simulink model "lab6_splp"  (R2023b)
settings: Solver=ode23t  StartTime=0.0  StopTime=Tmdl  MaxStep=1e-4  RelTol=1e-3
undefined symbols (not defined in the file): b0, b1, b2, Cm, crlp, Kd, Ki, Kp, R, To, Tur, w_target, X, Y, Z
libraries: sm_lib x12, fl_lib x7, nesl_utility x6, fl_ps_legacy_lib x2, ee_lib x1
settings Model: Creator=artur  LastModifiedBy=deniskirbaba
settings SolverCC: AlgebraicLoopSolver=TrustRegion
settings DataIOCC: ReturnWorkspaceOutputs=off
settings DebuggingCC: UnconnectedInputMsg=warning  UnconnectedOutputMsg=warning  UnconnectedLineMsg=warning  ArithmeticOperatorsInVariantConditions=warning
settings ModelReferenceCC: EnableRefExpFcnMdlSchedulingChecks=on
settings SFSimCC: SimUseLocalCustomCode=off  CustomCodeUndefinedFunction=UseInterfaceOnly
settings RTWCC: RTWUseLocalCustomCode=off
settings DiagnosticsConfigSet: SimMechanicsUnconnectedFramePorts=none  SimMechanicsUnconnectedGeometryPorts=none  SimMechanicsRigidlyBoundBlock=none

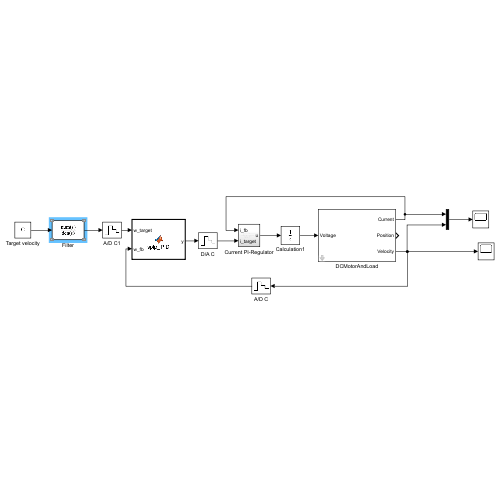
[thumbnail: Simulink's stored preview of the top-level diagram]
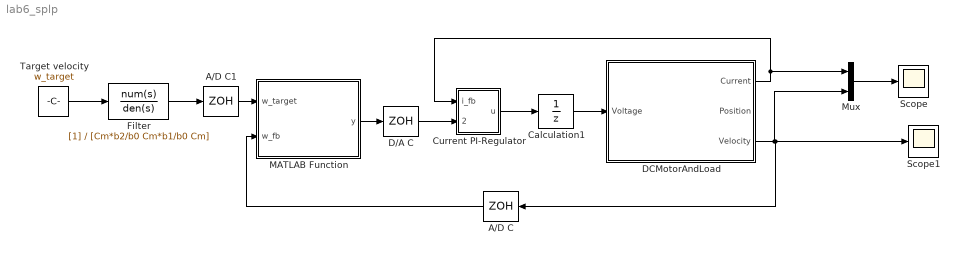
== system lab6_splp ==
  A/D C : ZeroOrderHold  SampleTime=To
  A/D C1 : ZeroOrderHold  SampleTime=To
  Calculation1 : UnitDelay  SampleTime=To/1000  HasFrameUpgradeWarning=on
  Current PI-Regulator : Subsystem
  D/A C : ZeroOrderHold  SampleTime=To
  DCMotorAndLoad : Subsystem  mask{PositionTargetValue=0, gain=0}
      mask prompts: PositionTargetValue "Position [deg]"; gain "Brakes (Off: 0, On: -1)"
      mask TypeOptions PositionTargetValue: Revolute1/PositionTargetValue
      mask TypeOptions gain: Brake/gain
      mask DialogControl Container3 Prompt: Parameters
  Filter : TransferFcn  Denominator=[Cm*b2/b0 Cm*b1/b0 Cm]
  MATLAB Function : MATLAB Function  TreatAsAtomicUnit=on
  Mux : Mux  Inputs=2
  Scope : Scope
  Scope1 : Scope
  Target velocity : Constant  Value=w_target
  wires:
  DCMotorAndLoad/1(Current) -> Current PI-Regulator/1(i_fb), Mux/1
  Mux/1 -> Scope/1
  Current PI-Regulator/1(u) -> Calculation1/1
  D/A C/1 -> Current PI-Regulator/2(i_target)
  DCMotorAndLoad/3(Velocity) -> Mux/2, A/D C/1, Scope1/1
  Calculation1/1 -> DCMotorAndLoad/1(Voltage)
  A/D C/1 -> MATLAB Function/2(w_fb)
  Target velocity/1 -> Filter/1
  Filter/1 -> A/D C1/1
  A/D C1/1 -> MATLAB Function/1(w_target)
  MATLAB Function/1(y) -> D/A C/1

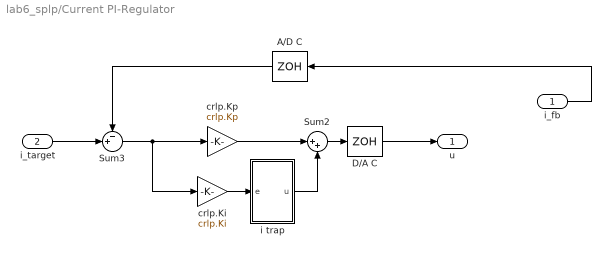
== system lab6_splp/Current PI-Regulator ==
  i_fb : Inport
  i_target : Inport  Port=2
  A/D C : ZeroOrderHold  SampleTime=To
  D/A C : ZeroOrderHold  SampleTime=To
  Sum2 : Sum  Inputs=|++
  Sum3 : Sum  Inputs=-+|
  crlp.Ki : Gain  Gain=crlp.Ki
  crlp.Kp : Gain  Gain=crlp.Kp
  i trap : Subsystem
  u : Outport
  wires:
  Sum3/1 -> crlp.Ki/1, crlp.Kp/1
  Sum2/1 -> D/A C/1
  i trap/1(u) -> Sum2/2
  crlp.Ki/1 -> i trap/1(e)
  A/D C/1 -> Sum3/1
  D/A C/1 -> u/1
  crlp.Kp/1 -> Sum2/1
  i_fb/1 -> A/D C/1
  i_target/1 -> Sum3/2

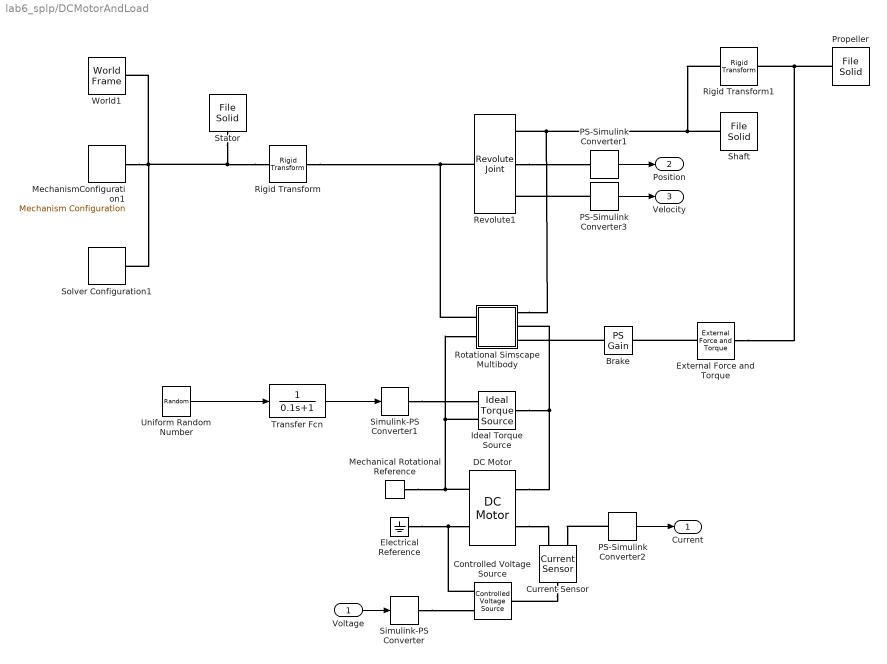
== system lab6_splp/DCMotorAndLoad ==
  Voltage : Inport
  Brake : fl_ps_legacy_lib/Legacy Physical Signals/Functions/PS Gain  gain=gain
  Controlled Voltage Source : fl_lib/Electrical/Electrical Sources/Controlled Voltage Source
  Current Sensor : fl_lib/Electrical/Electrical Sensors/Current Sensor
  DC Motor : ee_lib/Electromechanical/Brushed Motors/DC Motor  field_option=ee.enum.field_option.pm  Rf=100 Ohm  Lf=1 H  Laf=0.15 H  If0=0 A  parameterization=1  Ra=R Ohm  La=L H  emf_or_torque=1  Kv=Ce V/(rad/s)  Ki=R N*m/A  T_stall=0.24e-3 N*m  w_max=19100 rpm  w_rated=15000 rpm  P_rated=0.08 W  V_rated=1.5 V  lam_param=1  i_noload=0 A  V_i_noload=1.5 V  J=0 kg*m^2  lam=0 N*m/(rad/s)  speed0=0 rpm  enable_fault_armature=simscape.enum.onoff.off  rev_faulted=1 / 3  G_faulted_armature=1e-5 S  fault_trigger_armature=ee.enum.faults.faultTrigger.temporal  t_fault_armature=1 s  max_permissible_current_armature=inf A  t_fail_on_current_armature=1 s  enable_fault_field=simscape.enum.onoff.off  G_faulted_field=1e-5 S  fault_trigger_field=ee.enum.faults.faultTrigger.temporal  t_fault_field=1 s  max_permissible_current_field=inf A  t_fail_on_current_field=1 s  fault_action=simscape.enum.assert.action.none  alpha=3.93e-3 1/K  Tmeas=25 degC  thermal_mass=100 J/K  initial_temperature=25 degC
  Electrical Reference : fl_lib/Electrical/Electrical Elements/Electrical Reference
  External Force and Torque : sm_lib/Forces and Torques/External Force and Torque  ForceResolutionFrame=AttachedFrame  EnableForceX=off  EnableForceY=off  EnableForceZ=off  EnableForce=off  TorqueResolutionFrame=AttachedFrame  EnableTorqueX=off  EnableTorqueY=off  EnableTorqueZ=on  EnableTorque=off
  Ideal Torque Source : fl_lib/Mechanical/Mechanical Sources/Ideal Torque Source
  Mechanical Rotational Reference : fl_lib/Mechanical/Rotational Elements/Mechanical Rotational Reference
  MechanismConfiguration1 : sm_lib/Utilities/Mechanism Configuration  UniformGravity=Constant  GravityVector=[0 0 0]  GravityVectorUnits=m/s^2  LinearizationDelta=0.001  JointModeTransitionNonlinearIterations=2
  PS-Simulink Converter1 : nesl_utility/PS-Simulink Converter  PhysicalDomain=network_engine_domain  SubClassName=ps_output  LeftPortType=input  RightPortType=output  PseudoPeriodic=off  Frequencies=[]  VectorFormat=1-D array  Unit=1  AffineConversion=off
  PS-Simulink Converter2 : nesl_utility/PS-Simulink Converter  PhysicalDomain=network_engine_domain  SubClassName=ps_output  LeftPortType=input  RightPortType=output  PseudoPeriodic=off  Frequencies=[]  VectorFormat=1-D array  Unit=1  AffineConversion=off
  PS-Simulink Converter3 : nesl_utility/PS-Simulink Converter  PhysicalDomain=network_engine_domain  SubClassName=ps_output  LeftPortType=input  RightPortType=output  PseudoPeriodic=off  Frequencies=[]  VectorFormat=1-D array  Unit=deg/s  AffineConversion=off
  Propeller : sm_lib/Body Elements/File Solid  ExtGeomFileName=Propeller1_Default_sldprt.STEP  UnitType=FromFile  ExtGeomFileUnits=m  StepReaderType=HEX  ExportConvexHullGeometry=off  InertiaType=Custom  Mass=2.3673728265839591  MassUnits=kg  CenterOfMass=[0.0032690420415112924 -0.011715514211540433 5.1172052005901403]  CenterOfMassUnits=mm  MomentsOfInertia=[35196.968191955428 35197.433993512022 69961.334720373474]  MomentsOfInertiaUnits=kg*mm^2  ProductsOfInertia=[0.37928312011877774 -0.26254151093202421 1.2068537582504095]  ProductsOfInertiaUnits=kg*mm^2  BasedOnType=Density  Density=1000  DensityUnits=kg/m^3  DoExposeReferenceFrame=on  SerializedFrames=<Frames/>  GraphicType=FromGeometry  MarkerShape=Sphere  MarkerSize=10  GraphicVisPropType=SimpleVisualProperties  GraphicDiffuseColor=[1.0 1.0 1.0]  GraphicSpecularColor=[0.5 0.5 0.5 1.0]  GraphicAmbientColor=[0.15 0.15 0.15 1.0]  GraphicEmissiveColor=[0.0 0.0 0.0 1.0]  GraphicShininess=0  GraphicOpacity=1
  Revolute1 : sm_lib/Joints/Revolute Joint  JointMode=Normal  SenseConstraintForce=off  SenseConstraintForceX=off  SenseConstraintForceY=off  SenseConstraintForceZ=off  SenseConstraintTorque=off  SenseConstraintTorqueX=off  SenseConstraintTorqueY=off  SenseConstraintTorqueZ=off  SenseTotalForce=off  SenseTotalForceX=off  SenseTotalForceY=off  SenseTotalForceZ=off  SenseTotalTorque=off  SenseTotalTorqueX=off  SenseTotalTorqueY=off  SenseTotalTorqueZ=off  CompositeWrenchDir=FollowerOnBase  CompositeWrenchFrame=BaseFrame  EquilibriumPosition=0  EquilibriumPositionUnits=rad  SpringStiffness=0  SpringStiffnessUnits=N*m/rad  DampingCoefficient=0  DampingCoefficientUnits=N*m/(rad/s)  TorqueActuationMode=NoTorque  MotionActuationMode=ComputedMotion  SensePosition=on  SenseVelocity=on  SenseAcceleration=off  SenseTorqueForce=off  SenseLowerLimitTorqueForce=off  SenseUpperLimitTorqueForce=off  LowerLimitSpecify=off  LowerLimitBound=-90  LowerLimitBoundUnits=deg  LowerLimitStiffness=1e4  LowerLimitStiffnessUnits=N*m/deg  LowerLimitDamping=10  LowerLimitDampingUnits=N*m/(deg/s)  LowerLimitTransitionRegionWidth=0.1  LowerLimitTransitionRegionWidthUnits=deg  UpperLimitSpecify=off  UpperLimitBound=90  UpperLimitBoundUnits=deg  UpperLimitStiffness=1e4  UpperLimitStiffnessUnits=N*m/deg  UpperLimitDamping=10  UpperLimitDampingUnits=N*m/(deg/s)  UpperLimitTransitionRegionWidth=0.1  UpperLimitTransitionRegionWidthUnits=deg  PositionTargetSpecify=on  PositionTargetPriority=Low  PositionTargetValue=PositionTargetValue  PositionTargetValueUnits=deg  VelocityTargetSpecify=off  VelocityTargetPriority=High  VelocityTargetValue=0  VelocityTargetValueUnits=deg/s
  Rigid Transform : sm_lib/Frames and Transforms/Rigid Transform  TranslationMethod=None  TranslationStandardOffset=0  TranslationStandardOffsetUnits=m  TranslationStandardAxis=+Z  TranslationCartesianOffset=[0 0 0]  TranslationCartesianOffsetUnits=m  TranslationROffset=0  TranslationROffsetUnits=m  TranslationZOffset=0  TranslationZOffsetUnits=m  TranslationThetaOffset=0  TranslationThetaOffsetUnits=deg  RotationMethod=StandardAxis  RotationAngleUnits=deg  RotationStandardAxis=+X  RotationAngle=90  RotationArbitraryAxis=[0 0 1]  FollAlignAxisA=+X  BaseAlignAxisA=+Y  FollAlignAxisB=+Y  BaseAlignAxisB=+Z  RotationSequenceAxes=FollowerAxes  RotationSequence=XYX  RotationSequenceAngles=[0 0 0]  RotationSequenceAnglesUnits=deg  RotationMatrix=[1 0 0; 0 1 0; 0 0 1]  Quaternion=[1 0 0 0]
  Rigid Transform1 : sm_lib/Frames and Transforms/Rigid Transform  TranslationMethod=Cartesian  TranslationStandardOffset=0  TranslationStandardOffsetUnits=mm  TranslationStandardAxis=+Z  TranslationCartesianOffset=[0 0 110+30]  TranslationCartesianOffsetUnits=mm  TranslationROffset=0  TranslationROffsetUnits=m  TranslationZOffset=0  TranslationZOffsetUnits=m  TranslationThetaOffset=0  TranslationThetaOffsetUnits=deg  RotationMethod=None  RotationAngleUnits=deg  RotationStandardAxis=+X  RotationAngle=-90  RotationArbitraryAxis=[0 0 1]  FollAlignAxisA=+X  BaseAlignAxisA=+Y  FollAlignAxisB=+Y  BaseAlignAxisB=+Z  RotationSequenceAxes=FollowerAxes  RotationSequence=XYX  RotationSequenceAngles=[0 0 0]  RotationSequenceAnglesUnits=deg  RotationMatrix=[1 0 0; 0 1 0; 0 0 1]  Quaternion=[1 0 0 0]
  Rotational Simscape Multibody : Subsystem
  Shaft : sm_lib/Body Elements/File Solid  ExtGeomFileName=ShaftAndLoad7_Default_sldprt.STEP  UnitType=FromFile  ExtGeomFileUnits=m  StepReaderType=HEX  ExportConvexHullGeometry=off  InertiaType=Custom  Mass=1.8353573493569195  MassUnits=kg  CenterOfMass=[0 0 18.640525320290077]  CenterOfMassUnits=mm  MomentsOfInertia=[8427.9062058436339 8427.9062058436339 343.32904817379813]  MomentsOfInertiaUnits=kg*mm^2  ProductsOfInertia=[0 0 0]  ProductsOfInertiaUnits=kg*mm^2  BasedOnType=Density  Density=1000  DensityUnits=kg/m^3  DoExposeReferenceFrame=on  SerializedFrames=<Frames/>  GraphicType=FromGeometry  MarkerShape=Sphere  MarkerSize=10  GraphicVisPropType=SimpleVisualProperties  GraphicDiffuseColor=[0.6470588235294118 0.61960784313725492 0.58823529411764708]  GraphicSpecularColor=[0.5 0.5 0.5 1.0]  GraphicAmbientColor=[0.15 0.15 0.15 1.0]  GraphicEmissiveColor=[0.0 0.0 0.0 1.0]  GraphicShininess=75  GraphicOpacity=1
  Simulink-PS Converter : nesl_utility/Simulink-PS Converter  PhysicalDomain=network_engine_domain  SubClassName=ps_input  LeftPortType=input  RightPortType=output  PseudoPeriodic=off  Frequencies=[]  NoiseDistribution=none  NoiseParameters=[]  Unit=V  AffineConversion=off  FilteringAndDerivatives=zero  SimscapeFilterOrder=2  InputFilterTimeConstant=0.001  UdotUserProvided=1
  Simulink-PS Converter1 : nesl_utility/Simulink-PS Converter  PhysicalDomain=network_engine_domain  SubClassName=ps_input  LeftPortType=input  RightPortType=output  PseudoPeriodic=off  Frequencies=[]  NoiseDistribution=none  NoiseParameters=[]  Unit=N*m  AffineConversion=off  FilteringAndDerivatives=zero  SimscapeFilterOrder=2  InputFilterTimeConstant=0.001  UdotUserProvided=1
  Solver Configuration1 : nesl_utility/Solver Configuration  PhysicalDomain=network_engine_domain  SubClassName=solver  LeftPortType=input  RightPortType=generic  Tones=[]  Harmonics=[]  SimulateNoise=off  Profile=off  UseLocalSampling=off  EnableSwitchedLinearOptims=on  FrequencyDomain=off  UseCCode=off  RelTol=0.001  AbsTol=1e-06  MinStep=1e-09  ToWorkspace=off  RevertToSquareIcSolve=off  NumHomotopyIterations=100  PhasorMode=off  PhasorModeNumHarmonics=1  ConsistencySolver=NEWTON_FTOL  IndexReductionMethod=DerivativeReplacement  DoDC=off  ResidualTolerance=1e-09  ConsistencyTolSource=GLOBAL  ConsistencyAbsTol=0.001  ConsistencyRelTol=0.001  ConsistencyTolFactor=0.001  UseLocalSolver=off  LocalSolverChoice=NE_BACKWARD_EULER_ADVANCER  ResolveIndetEquations=on  FunctionEvalNumThread=1  LocalSolverSampleTime=0.001  DoFixedCost=off  MaxNonlinIter=3  MaxModeIter=2  ComputeImpulses=off  ImpulseIterations=2  LinearAlgebra=Sparse  LinearAlgebraNumThread=0  EquationFormulation=NE_TIME_EF  DelaysMemoryBudget=1024  AutomaticFiltering=on  FilteringTimeConstant=0.001  PartitionStorageMethod=AS_NEEDED  PartitionMemoryBudget=1024  PartitionMethod=FAST  MultibodyUseLocalSolver=off  MultibodyLocalSolverChoice=ODE1  MultibodyLocalSolverSampleTime=0.001
  Stator : sm_lib/Body Elements/File Solid  ExtGeomFileName=Stator_Default_sldprt.STEP  UnitType=FromFile  ExtGeomFileUnits=m  StepReaderType=HEX  ExportConvexHullGeometry=off  InertiaType=Custom  Mass=29.434213631466882  MassUnits=kg  CenterOfMass=[5.0575987079983372e-05 0 -8.9565096724242519]  CenterOfMassUnits=mm  MomentsOfInertia=[149918.89673856943 102257.27891592759 136644.67697517879]  MomentsOfInertiaUnits=kg*mm^2  ProductsOfInertia=[0 0.081308539805349009 -0.0002124915132821191]  ProductsOfInertiaUnits=kg*mm^2  BasedOnType=Density  Density=1000  DensityUnits=kg/m^3  DoExposeReferenceFrame=on  SerializedFrames=<Frames/>  GraphicType=FromGeometry  MarkerShape=Sphere  MarkerSize=10  GraphicVisPropType=SimpleVisualProperties  GraphicDiffuseColor=[0.4 0.4 0.4]  GraphicSpecularColor=[0.5 0.5 0.5 1.0]  GraphicAmbientColor=[0.15 0.15 0.15 1.0]  GraphicEmissiveColor=[0.0 0.0 0.0 1.0]  GraphicShininess=1  GraphicOpacity=1
  Transfer Fcn : TransferFcn  Denominator=[0.1 1]
  Uniform Random Number : UniformRandomNumber  SampleTime=0.001
  World1 : sm_lib/Frames and Transforms/World Frame
  Current : Outport  VectorParamsAs1DForOutWhenUnconnected=off
  Position : Outport  Port=2  VectorParamsAs1DForOutWhenUnconnected=off
  Velocity : Outport  Port=3  VectorParamsAs1DForOutWhenUnconnected=off
  wires:
  Voltage/1 -> Simulink-PS Converter/1
  PS-Simulink Converter2/1 -> Current/1
  PS-Simulink Converter1/1 -> Position/1
  PS-Simulink Converter3/1 -> Velocity/1
  Transfer Fcn/1 -> Simulink-PS Converter1/1
  Uniform Random Number/1 -> Transfer Fcn/1
  connections:
  DC Motor/LConn2 -- Ideal Torque Source/LConn1 -- Rotational Simscape Multibody/RConn2
  DC Motor/RConn2 -- Mechanical Rotational Reference/LConn1 -- Ideal Torque Source/RConn2 -- Rotational Simscape Multibody/LConn2
  Controlled Voltage Source/RConn2 -- DC Motor/RConn1 -- Electrical Reference/LConn1
  Simulink-PS Converter/RConn1 -- Controlled Voltage Source/RConn1
  Rigid Transform/LConn1 -- Stator/RConn1 -- Solver Configuration1/RConn1 -- MechanismConfiguration1/RConn1 -- World1/RConn1
  DC Motor/LConn1 -- Current Sensor/RConn2
  Current Sensor/LConn1 -- Controlled Voltage Source/LConn1
  PS-Simulink Converter2/LConn1 -- Current Sensor/RConn1
  Revolute1/LConn1 -- Rigid Transform/RConn1 -- Rotational Simscape Multibody/LConn1
  Propeller/RConn1 -- External Force and Torque/RConn1 -- Rigid Transform1/RConn1
  Revolute1/RConn2 -- PS-Simulink Converter1/LConn1
  PS-Simulink Converter3/LConn1 -- Revolute1/RConn3
  Rigid Transform1/LConn1 -- Shaft/RConn1 -- Rotational Simscape Multibody/RConn1 -- Revolute1/RConn1
  Simulink-PS Converter1/RConn1 -- Ideal Torque Source/RConn1
  External Force and Torque/LConn1 -- Brake/RConn1
  Brake/LConn1 -- Rotational Simscape Multibody/RConn3

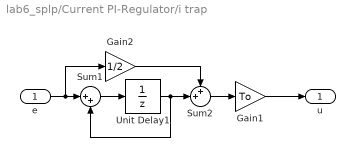
== system lab6_splp/Current PI-Regulator/i trap ==
  e : Inport
  Gain1 : Gain  Gain=To
  Gain2 : Gain  Gain=1/2
  Sum1 : Sum  Inputs=|++
  Sum2 : Sum  Inputs=++|
  Unit Delay1 : UnitDelay  SampleTime=To  HasFrameUpgradeWarning=on
  u : Outport
  wires:
  Unit Delay1/1 -> Sum2/2, Sum1/2
  Sum2/1 -> Gain1/1
  Gain2/1 -> Sum2/1
  Sum1/1 -> Unit Delay1/1
  e/1 -> Gain2/1, Sum1/1
  Gain1/1 -> u/1

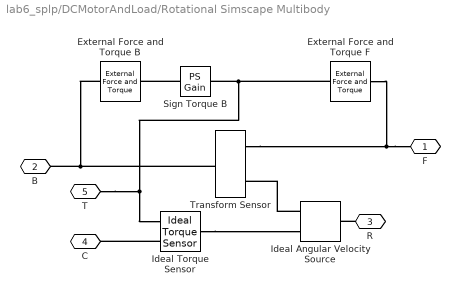
== system lab6_splp/DCMotorAndLoad/Rotational Simscape Multibody ==
  External Force and Torque B : sm_lib/Forces and Torques/External Force and Torque  ForceResolutionFrame=AttachedFrame  EnableForceX=off  EnableForceY=off  EnableForceZ=off  EnableForce=off  TorqueResolutionFrame=AttachedFrame  EnableTorqueX=off  EnableTorqueY=off  EnableTorqueZ=on  EnableTorque=off
  External Force and Torque F : sm_lib/Forces and Torques/External Force and Torque  ForceResolutionFrame=AttachedFrame  EnableForceX=off  EnableForceY=off  EnableForceZ=off  EnableForce=off  TorqueResolutionFrame=AttachedFrame  EnableTorqueX=off  EnableTorqueY=off  EnableTorqueZ=on  EnableTorque=off
  Ideal Angular Velocity Source : fl_lib/Mechanical/Mechanical Sources/Ideal Angular Velocity Source
  Ideal Torque Sensor : fl_lib/Mechanical/Mechanical Sensors/Ideal Torque Sensor
  Sign Torque B : fl_ps_legacy_lib/Legacy Physical Signals/Functions/PS Gain  gain=-1
  Transform Sensor : sm_lib/Frames and Transforms/Transform Sensor  MeasurementFrame=Base  RotationSequence=XYX  SenseAngle=off  SenseAxis=off  SenseQ=off  SenseR=off  SenseRotationSequence=off  SenseOmegaX=off  SenseOmegaY=off  SenseOmegaZ=on  SenseOmega=off  SenseQDot=off  SenseRDot=off  SenseRotationSequenceDot=off  SenseAlphaX=off  SenseAlphaY=off  SenseAlphaZ=off  SenseAlpha=off  SenseQDDot=off  SenseRDDot=off  SenseX=off  SenseY=off  SenseZ=off  SenseXYZ=off  SenseRad=off  SenseAzim=off  SenseDist=off  SenseInc=off  SenseXDot=off  SenseYDot=off  SenseZDot=off  SenseXYZDot=off  SenseRadDot=off  SenseAzimDot=off  SenseDistDot=off  SenseIncDot=off  SenseXDDot=off  SenseYDDot=off  SenseZDDot=off  SenseXYZDDot=off  SenseRadDDot=off  SenseAzimDDot=off  SenseDistDDot=off  SenseIncDDot=off
  F : PMIOPort  Side=Right
  B : PMIOPort  Port=2  Side=Left
  R : PMIOPort  Port=3  Side=Right
  C : PMIOPort  Port=4  Side=Left
  T : PMIOPort  Port=5  Side=Right
  connections:
  Sign Torque B/LConn1 -- T/RConn1 -- Ideal Torque Sensor/RConn2 -- External Force and Torque F/LConn1
  Sign Torque B/RConn1 -- External Force and Torque B/LConn1
  Ideal Angular Velocity Source/RConn1 -- Transform Sensor/RConn2
  F/RConn1 -- External Force and Torque F/RConn1 -- Transform Sensor/RConn1
  External Force and Torque B/RConn1 -- B/RConn1 -- Transform Sensor/LConn1
  Ideal Torque Sensor/LConn1 -- Ideal Angular Velocity Source/RConn2
  R/RConn1 -- Ideal Angular Velocity Source/LConn1
  Ideal Torque Sensor/RConn1 -- C/RConn1

== matlab function lab6_splp/MATLAB Function ==
  data: y output; w_target input; w_fb input; To parameter; Tur parameter; Kp parameter; Ki parameter; Kd parameter
function y = splp_PID(w_target, w_fb, To, Tur, Kp, Ki, Kd)

persistent u_old e_old ud
if isempty(u_old)
    u_old = 0;
    e_old = 0;
    ud = 0;
end

e = w_target - w_fb;
u = u_old + (e + e_old)*Ki*To/2;
ud = 1/(To + 2*Tur)*(2*(e - e_old) - (To - 2*Tur)*ud);
y = Kp*e + u + Kd*ud;

u_old = u;
e_old = e;
